simulink model "fitz_relay_added_current"  (R2015a)
settings: Solver=ode45  StartTime=0.0  StopTime=tmax  RelTol=1e-3
values from neighbouring files (symbols this model uses):
  A = gamma-alpha    (= 2.5)    [added_current_fitz_relay.m]    (also in example_1.m = [0 1 1; 0 -1 6; 0 0 -1]; getAsymmetricRelayHysteresisForFitzNagumo.m = -0.5; goodwin_prediction.m = [-1 0 0 ; 1 -1 0; 0 1 -1]; new_fitz_relay.m = -1.5)
  d2 = 0.25    [added_current_fitz_relay.m]    (also in epsilon_sensitivity_to_d1_d2.m = 0.2829; goodwin_prediction.m = 0; new_fitz_relay.m; relay_fitz_nagumo.m = abs(mean([a(2,2) a(2,4)])))
  epsilon_1 = out(1)    [added_current_fitz_relay.m]    (also in example_1.m = -1; new_fitz_relay.m = -(epsilon_1 - I_app); relay_fitz_nagumo.m = a(1,1))
  epsilon_2 = out(2)    [added_current_fitz_relay.m]    (also in example_1.m = 1; new_fitz_relay.m = -(epsilon_2 - I_app); relay_fitz_nagumo.m = a(1,3))
  X0 = a1    [added_current_fitz_relay.m]    (also in example_1.m; new_fitz_relay.m; relay_fitz_nagumo.m = a2; test_goodwin.m = -a1)
settings Model: Creator=ra428  LastModifiedBy=ra428

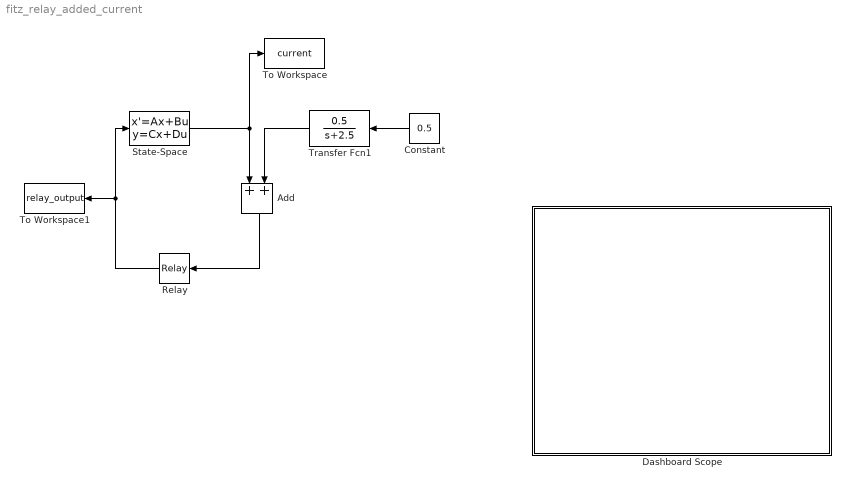
== system fitz_relay_added_current ==
  Add : Sum
  Constant : Constant  Value=0.5
  Dashboard Scope : Subsystem  DialogController=hmiCreateDDGDialog  IsWebBlock=on  mask(MathWorksWebBlock){webBlockId=43bc493d-58c7-4b0c-93af-8cc9f44ef554, webBlockType=sdiscope, ShowInitialText=on, HMISrcModelName=fitz_relay_added_current}
      mask prompts: webBlockId "WebBlock Id"; webBlockType "WebBlock Type"; HMISrcModelName "Source Model"
      mask Help: helpview([docroot '/mapfiles/simulink.map'], 'hmi_scope')
      mask Display:
      | if strcmp(get_param(bdroot(gcb),'BlockDiagramType'), 'library')
      |     image([(matlabroot) '/toolbox/simulink/hmi/icons/DashboardScope.png']);
      | end
  Relay : Relay  OnSwitchValue=epsilon_2  OffSwitchValue=epsilon_1  OnOutputValue=-d2  OffOutputValue=d1
  State-Space : StateSpace  A=A  D=0  X0=X0
  To Workspace : ToWorkspace  VariableName=current  SaveFormat=Timeseries  SampleTime=-1
  To Workspace1 : ToWorkspace  VariableName=relay_output  SaveFormat=Timeseries  SampleTime=-1
  Transfer Fcn1 : TransferFcn  Numerator=[0.5]  Denominator=[1 2.5]
  wires:
  Transfer Fcn1/1 -> Add/2
  Add/1 -> Relay/1
  Constant/1 -> Transfer Fcn1/1
  State-Space/1 -> Add/1, To Workspace/1
  Relay/1 -> State-Space/1, To Workspace1/1

== system fitz_relay_added_current/Dashboard Scope ==
